simulink library "PESRC01MSEREF"  (R2014b)
settings: Solver=ode45  StartTime=0.0  StopTime=10.0  RelTol=1e-3
undefined symbols (not defined in the file): errordlg
libraries: simulink x27
settings Model: Creator=vda2sh  LastModifiedBy=RUS1COB

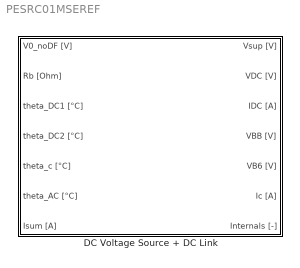
== system PESRC01MSEREF ==
  DC Voltage Source + DC Link : Subsystem  Tag=PESRC01MSEREF  mask(PESRC01MSEREF){Lb=5e-6, Cb=1, RDC120=5e-3, alphaDC1=0, RDC220=1e-3, alphaDC2=0, LDC2=4e-5, C=600e-6, Rc20=1e-3, alphac=0, RAC20=1e-3, alphaAC=0, IDC_init=0, qDC_init=0, Vc_init=0}
      mask prompts: Lb "DC voltage source internal inductance [H]"; Cb "DC voltage source capacity [Ah]"; RDC120 "Wire harness resistance at 20°C [Ohm]"; alphaDC1 "Thermal coefficient of wire harness resistance [1/K]"; RDC220 "Power net resistance at 20°C [Ohm]"; alphaDC2 "Thermal coefficient of power net resistance [1/K]"; LDC2 "Power net inductance [H]"; C "DC-link capacitor [F]"; Rc20 "DC-link resistance at 20°C [Ohm]"; alphac "Thermal coefficient of DC-link resistance [1/K]"; RAC20 "Cable resistance between DC-link and drive at 20°C [Ohm]"; alphaAC "Thermal coefficient of cable resistance between DC-link and drive [1/K]"; IDC_init "Initial DC voltage source current (case Lb+LDC2>0) [A]"; qDC_init "Initial DC voltage source charge [C]"; Vc_init "Initial DC-link capacitor voltage [V]"
      mask help:
      | PESRC01MSEREF - DC Voltage Source and DC-Link Model
      |
      | This is a model of a DC voltage source connected a DC-link considering simple wire harness and power net effects.
      settings: AttributesFormatString=<%<Tag>>
      mask Help: eval('show_docs_mseref_powerelectronics(''PESRC01MSEREF'')')
      mask Display:
      | image(imread('PESRC01MSEREF.png'),[0.25, 0.25, 0.6, 0.6]);
      | text(0.6,0.15, 'MSE')
      | port_label('input',1,'V0_NoDF [V]')
      | port_label('input',2,'Rb [Ohm]')
      | port_label('input',3,'theta_DC1 [°C]')
      | port_label('input',4,'theta_DC2 [°C]')
      | port_label('input',5,'theta_c [°C]')
      | port_label('input',6,'theta_AC [°C]')
      | port_label('input',7,'Isum [A]')
      | port_label('output',1,'Vsup [V]')
      | port_label('output',2,'VDC [V]')
      | port_label('output',3,'IDC [A]')
      | port_label('output',4,'VBB [V]')
      | port_label('output',5,'VB6 [V]')
      | port_label('output',6,'Ic [A]')
      | port_label('output',7,'Internals')

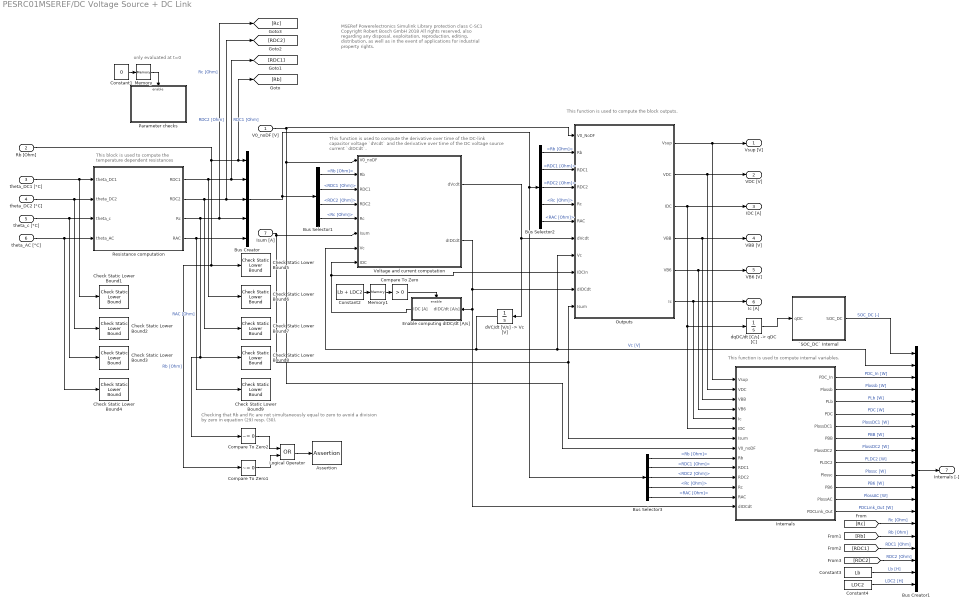
== system PESRC01MSEREF/DC Voltage Source + DC Link ==
  note: Checking that Rb and Rc are not simultaneously equal to zero to avoid
      | a division by zero in equation (29) resp. (30).
  note: This function is used to compute internal variables.
  note: This function is used to compute the block outputs.
  note: This function is used to compute the derivative over time
      | of the DC-link capacitor voltage `dVcdt`
      | and the derivative over time of the DC voltage source current `dIDCdt`.
  note: This block is used to compute
      | the temperature dependent resistances
  note: MSERef Powerelectronics Simulink Library
      | protection class C-SC1
      |
      | Copyright Robert Bosch GmbH 2018
      |
      | All rights reserved, also regarding any disposal, exploitation,
      | reproduction, editing, distribution, as well as in the event of
      | applications for industrial property rights.
  note: only evaluated at t=0
  V0_noDF [V] : Inport
  Rb [Ohm] : Inport  Port=2
  theta_DC1 [°C] : Inport  Port=3
  theta_DC2 [°C] : Inport  Port=4
  theta_c [°C] : Inport  Port=5
  theta_AC [°C] : Inport  Port=6
  Isum [A] : Inport  Port=7
  Assertion : Assertion  AssertionFailFcn=errordlg('ERROR: `DC voltage source internal resistance` Rb and `DC-link resistance`Rc(theta_c) are simultaneously equal to zero.')
  Bus Creator : BusCreator  Inputs=5
  Bus Creator1 : BusCreator  Inputs=20
  Bus Selector1 : BusSelector  OutputSignals=Rb [Ohm],RDC1 [Ohm],RDC2 [Ohm],Rc [Ohm]
  Bus Selector2 : BusSelector  OutputSignals=Rb [Ohm],RDC1 [Ohm],RDC2 [Ohm],Rc [Ohm],RAC [Ohm]
  Bus Selector3 : BusSelector  OutputSignals=Rb [Ohm],RDC1 [Ohm],RDC2 [Ohm],Rc [Ohm],RAC [Ohm]
  Check Static Lower Bound1 : simulink/Model Verification/Check Static  Lower Bound  Description=-273.15 < u  min=-273.15  min_included=off  enabled=on  callback=errordlg('Input `Wire harness temperature` theta_DC1 lower or equal to -273.15°C.')  stopWhenAssertionFail=on  export=off  icon=graphic
  Check Static Lower Bound2 : simulink/Model Verification/Check Static  Lower Bound  Description=-273.15 < u  min=-273.15  min_included=off  enabled=on  callback=errordlg('Input `Power net temperature` theta_DC2 lower or equal to -273.15°C.')  stopWhenAssertionFail=on  export=off  icon=graphic
  Check Static Lower Bound3 : simulink/Model Verification/Check Static  Lower Bound  Description=-273.15 < u  min=-273.15  min_included=off  enabled=on  callback=errordlg('Input `DC-link temperature` theta_c lower or equal to -273.15°C.')  stopWhenAssertionFail=on  export=off  icon=graphic
  Check Static Lower Bound4 : simulink/Model Verification/Check Static  Lower Bound  Description=-273.15 < u  min=-273.15  min_included=off  enabled=on  callback=errordlg('Input `Cable (between DC-link and drive) temperature` theta_AC lower or equal to -273.15°C.')  stopWhenAssertionFail=on  export=off  icon=graphic
  Check Static Lower Bound5 : simulink/Model Verification/Check Static  Lower Bound  Description=0 <= u  min=0  min_included=on  enabled=on  callback=errordlg('ERROR: `DC voltage source internal resistance` Rb is lower than zero.')  stopWhenAssertionFail=on  export=off  icon=graphic
  Check Static Lower Bound6 : simulink/Model Verification/Check Static  Lower Bound  Description=0 <= u  min=0  min_included=on  enabled=on  callback=errordlg('ERROR: `Wire harness resistance` RDC1(theta_DC1) is lower than zero.')  stopWhenAssertionFail=on  export=off  icon=graphic
  Check Static Lower Bound7 : simulink/Model Verification/Check Static  Lower Bound  Description=0 <= u  min=0  min_included=on  enabled=on  callback=errordlg('ERROR: `Power net resistance`RDC2(theta_DC2) is lower than zero.')  stopWhenAssertionFail=on  export=off  icon=graphic
  Check Static Lower Bound8 : simulink/Model Verification/Check Static  Lower Bound  Description=0 <= u  min=0  min_included=on  enabled=on  callback=errordlg('ERROR: `DC-link resistance`Rc(theta_c) is lower than zero.')  stopWhenAssertionFail=on  export=off  icon=graphic
  Check Static Lower Bound9 : simulink/Model Verification/Check Static  Lower Bound  Description=0 <= u  min=0  min_included=on  enabled=on  callback=errordlg('ERROR: `Cable resistance between DC-link and drive`RAC(theta_AC) is lower than zero.')  stopWhenAssertionFail=on  export=off  icon=graphic
  Compare To Zero : simulink/Logic and Bit Operations/Compare To Zero  relop=>  OutDataTypeStr=boolean
  Compare To Zero1 : simulink/Logic and Bit Operations/Compare To Zero  relop=~=  OutDataTypeStr=boolean
  Compare To Zero2 : simulink/Logic and Bit Operations/Compare To Zero  relop=~=  OutDataTypeStr=boolean
  Constant1 : Constant  Value=0
  Constant2 : Constant  Value=Lb + LDC2
  Constant3 : Constant  Value=Lb
  Constant4 : Constant  Value=LDC2
  Enable computing dIDC/dt [A/s] : Subsystem  TreatAsAtomicUnit=on
  Internals : MATLAB Function  TreatAsAtomicUnit=on
  Logical Operator : Logic  Operator=OR  AllPortsSameDT=off  OutDataTypeStr=boolean
  Memory : Memory  X0=1
  Memory1 : Memory  X0=1
  Outputs : MATLAB Function  TreatAsAtomicUnit=on
  Parameter checks : Subsystem
  Resistance computation : MATLAB Function  TreatAsAtomicUnit=on
  Voltage and current computation : MATLAB Function  TreatAsAtomicUnit=on
  `SOC_DC` Internal : MATLAB Function  TreatAsAtomicUnit=on
  "dVC/dt [V/s] -> Vc [V]" : Integrator  InitialCondition=Vc_init
  "dqDC/dt [C/s] -> qDC [C]" : Integrator  InitialCondition=qDC_init
  Vsup [V] : Outport
  VDC [V] : Outport  Port=2
  IDC [A] : Outport  Port=3
  VBB [V] : Outport  Port=4
  VB6 [V] : Outport  Port=5
  Ic [A] : Outport  Port=6
  Internals [-] : Outport  Port=7
  wires:
  Internals/7(PlossDC2) -> Bus Creator1/9  "PlossDC2 [W]"
  Internals/5(PlossDC1) -> Bus Creator1/7  "PlossDC1 [W]"
  Internals/9(Plossc) -> Bus Creator1/11  "Plossc [W]"
  Internals/3(PLb) -> Bus Creator1/5  "PLb [W]"
  Internals/11(PlossAC) -> Bus Creator1/13  "PlossAC [W]"
  Internals/12(PDCLink_Out) -> Bus Creator1/14  "PDCLink_Out [W]"
  Internals/8(PLDC2) -> Bus Creator1/10  "PLDC2 [W]"
  Internals/2(Plossb) -> Bus Creator1/4  "Plossb [W]"
  Internals/1(PDC_In) -> Bus Creator1/3  "PDC_In [W]"
  Bus Creator1/1 -> Internals [-]/1
  "dVC/dt [V/s] -> Vc [V]"/1 -> Voltage and current computation/7(Vc), Outputs/8(Vc), Bus Creator1/2  "Vc [V]"
  Bus Selector2/4 -> Outputs/5(Rc)  "<Rc [Ohm]>"
  Bus Selector2/2 -> Outputs/3(RDC1)  "<RDC1 [Ohm]>"
  Bus Selector3/2 -> Internals/10(RDC1)  "<RDC1 [Ohm]>"
  Bus Selector3/4 -> Internals/12(Rc)  "<Rc [Ohm]>"
  Bus Selector3/1 -> Internals/9(Rb)  "<Rb [Ohm]>"
  Bus Selector3/5 -> Internals/13(RAC)  "<RAC [Ohm]>"
  Bus Selector3/3 -> Internals/11(RDC2)  "<RDC2 [Ohm]>"
  Bus Selector2/1 -> Outputs/2(Rb)  "<Rb [Ohm]>"
  Bus Selector1/4 -> Voltage and current computation/5(Rc)  "<Rc [Ohm]>"
  Bus Selector1/3 -> Voltage and current computation/4(RDC2)  "<RDC2 [Ohm]>"
  Bus Selector1/2 -> Voltage and current computation/3(RDC1)  "<RDC1 [Ohm]>"
  Bus Selector1/1 -> Voltage and current computation/2(Rb)  "<Rb [Ohm]>"
  Bus Creator/1 -> Bus Selector1/1, Bus Selector3/1, Bus Selector2/1
  Resistance computation/4(RAC) -> Check Static Lower Bound9/1, Bus Creator/5  "RAC [Ohm]"
  Resistance computation/1(RDC1) -> Check Static Lower Bound6/1, [RDC1], Bus Creator/2  "RDC1 [Ohm]"
  Resistance computation/2(RDC2) -> Check Static Lower Bound7/1, [RDC2], Bus Creator/3  "RDC2 [Ohm]"
  theta_AC [°C]/1 -> Check Static Lower Bound4/1, Resistance computation/4(theta_AC)
  theta_c [°C]/1 -> Check Static Lower Bound3/1, Resistance computation/3(theta_c)
  theta_DC2 [°C]/1 -> Check Static Lower Bound2/1, Resistance computation/2(theta_DC2)
  theta_DC1 [°C]/1 -> Check Static Lower Bound1/1, Resistance computation/1(theta_DC1)
  Outputs/1(Vsup) -> Internals/1(Vsup), Vsup [V]/1
  Voltage and current computation/1(dVcdt) -> Outputs/7(dVcdt), "dVC/dt [V/s] -> Vc [V]"/1
  Isum [A]/1 -> Outputs/11(Isum), Internals/7(Isum), Voltage and current computation/6(Isum)
  Voltage and current computation/2(dIDCdt) -> Enable computing dIDC/dt [A/s]/1(dIDC/dt [A/s]), Internals/14(dIDCdt), Outputs/10(dIDCdt)
  Outputs/2(VDC) -> VDC [V]/1, Internals/2(VDC)
  Outputs/3(IDC) -> IDC [A]/1, Internals/6(IDC), "dqDC/dt [C/s] -> qDC [C]"/1
  Outputs/4(VBB) -> Internals/3(VBB), VBB [V]/1
  Outputs/5(VB6) -> Internals/4(VB6), VB6 [V]/1
  Outputs/6(Ic) -> Internals/5(Ic), Ic [A]/1
  Constant1/1 -> Memory/1
  Memory/1 -> Parameter checks/Enable
  V0_noDF [V]/1 -> Voltage and current computation/1(V0_noDF), Internals/8(V0_noDF), Outputs/1(V0_NoDF)
  Internals/10(PB6) -> Bus Creator1/12  "PB6 [W]"
  Internals/6(PBB) -> Bus Creator1/8  "PBB [W]"
  Internals/4(PDC) -> Bus Creator1/6  "PDC [W]"
  Enable computing dIDC/dt [A/s]/1(IDC [A]) -> Outputs/9(IDCIn), Voltage and current computation/8(IDC)
  Bus Selector2/5 -> Outputs/6(RAC)  "<RAC [Ohm]>"
  Bus Selector2/3 -> Outputs/4(RDC2)  "<RDC2 [Ohm]>"
  Compare To Zero/1 -> Enable computing dIDC/dt [A/s]/Enable
  Memory1/1 -> Compare To Zero/1
  Constant2/1 -> Memory1/1
  Compare To Zero2/1 -> Logical Operator/1
  Compare To Zero1/1 -> Logical Operator/2
  Logical Operator/1 -> Assertion/1
  `SOC_DC` Internal/1(SOC_DC) -> Bus Creator1/1  "SOC_DC [-]"
  "dqDC/dt [C/s] -> qDC [C]"/1 -> `SOC_DC` Internal/1(qDC)
  Resistance computation/3(Rc) -> Compare To Zero2/1, Check Static Lower Bound8/1, [Rc], Bus Creator/4  "Rc [Ohm]"
  Rb [Ohm]/1 -> Compare To Zero1/1, Check Static Lower Bound5/1, [Rb], Bus Creator/1  "Rb [Ohm]"
  [Rc] -> Bus Creator1/15  "Rc [Ohm]"
  [Rb] -> Bus Creator1/16  "Rb [Ohm]"
  [RDC1] -> Bus Creator1/17  "RDC1 [Ohm]"
  [RDC2] -> Bus Creator1/18  "RDC2 [Ohm]"
  Constant3/1 -> Bus Creator1/19  "Lb [H]"
  Constant4/1 -> Bus Creator1/20  "LDC2 [H]"

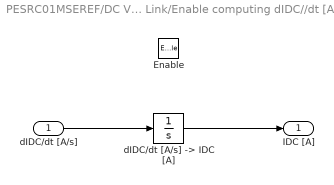
== system PESRC01MSEREF/DC Voltage Source + DC Link/Enable computing dIDC//dt [A//s] ==
  dIDC/dt [A/s] : Inport
  Enable : EnablePort
  "dIDC/dt [A/s] -> IDC [A]" : Integrator  InitialCondition=IDC_init
  IDC [A] : Outport
  wires:
  dIDC/dt [A/s]/1 -> "dIDC/dt [A/s] -> IDC [A]"/1
  "dIDC/dt [A/s] -> IDC [A]"/1 -> IDC [A]/1

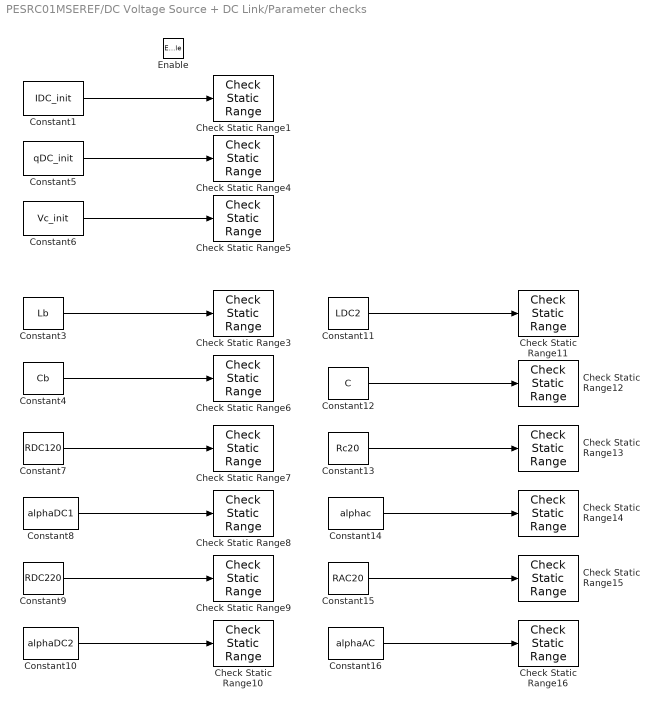
== system PESRC01MSEREF/DC Voltage Source + DC Link/Parameter checks ==
  Enable : EnablePort  ZeroCross=off
  Check Static Range1 : simulink/Model Verification/Check  Static Range  Description=-1e9 <= u < 1e9  max=1e9  max_included=off  min=-1e9  min_included=on  enabled=on  callback=errordlg('Parameter `Initial DC voltage source current` IDC_init outside boundary [-1e9, 1e9] A.')  stopWhenAssertionFail=on  export=off  icon=graphic
  Check Static Range10 : simulink/Model Verification/Check  Static Range  Description=0 <= u <= 1  max=1  max_included=on  min=0  min_included=on  enabled=on  callback=errordlg('Parameter `Thermal coefficient of power net resistance` alphaDC1 outside boundary [0, 1] 1/K.')  stopWhenAssertionFail=on  export=off  icon=graphic
  Check Static Range11 : simulink/Model Verification/Check  Static Range  Description=0 <= u <= 10  max=10  max_included=on  min=0  min_included=on  enabled=on  callback=errordlg('Parameter `Power net inductance` LDC2 outside boundary [0, 10] H.')  stopWhenAssertionFail=on  export=off  icon=graphic
  Check Static Range12 : simulink/Model Verification/Check  Static Range  Description=0 <= u <= 1e3  max=1e3  max_included=on  min=0  min_included=on  enabled=on  callback=errordlg('Parameter `DC-link capacitor` C outside boundary [0, 1e3] F.')  stopWhenAssertionFail=on  export=off  icon=graphic
  Check Static Range13 : simulink/Model Verification/Check  Static Range  Description=0 <= u <= 1e9  max=1e9  max_included=on  min=0  min_included=on  enabled=on  callback="errordlg('Parameter `DC-link resistance  at 20°C` Rc20 outside boundary ]0, 1e9] Ohm.')"  stopWhenAssertionFail=on  export=off  icon=graphic
  Check Static Range14 : simulink/Model Verification/Check  Static Range  Description=0 <= u <= 1  max=1  max_included=on  min=0  min_included=on  enabled=on  callback=errordlg('Parameter `Thermal coefficient of DC-link resistance` alphac outside boundary [0, 1] 1/K.')  stopWhenAssertionFail=on  export=off  icon=graphic
  Check Static Range15 : simulink/Model Verification/Check  Static Range  Description=0 <= u <= 1e9  max=1e9  max_included=on  min=0  min_included=on  enabled=on  callback=errordlg('Parameter `Cable resistance between DC-link and drive at 20°C` RAC20 outside boundary [0, 1e9] Ohm.')  stopWhenAssertionFail=on  export=off  icon=graphic
  Check Static Range16 : simulink/Model Verification/Check  Static Range  Description=0 <= u <= 1  max=1  max_included=on  min=0  min_included=on  enabled=on  callback=errordlg('Parameter `Thermal coefficient of cable resistance between DC-link and drive` alphaAC outside boundary [0, 1] 1/K.')  stopWhenAssertionFail=on  export=off  icon=graphic
  Check Static Range3 : simulink/Model Verification/Check  Static Range  Description=0 <= u <= 10  max=10  max_included=on  min=0  min_included=on  enabled=on  callback=errordlg('Parameter `DC voltage source internal inductance` Lb outside boundary [0, 10] H.')  stopWhenAssertionFail=on  export=off  icon=graphic
  Check Static Range4 : simulink/Model Verification/Check  Static Range  Description=-1e9 <= u < 1e9  max=1e9  max_included=off  min=-1e9  min_included=on  enabled=on  callback=errordlg('Parameter `Initial DC voltage source charge` qDC_init outside boundary [-1e9, 1e9] C.')  stopWhenAssertionFail=on  export=off  icon=graphic
  Check Static Range5 : simulink/Model Verification/Check  Static Range  Description=-1e9 <= u < 1e9  max=1e9  max_included=off  min=-1e9  min_included=on  enabled=on  callback=errordlg('Parameter `Initial DC-link capacitor voltage` Vc_init outside boundary [-1e9, 1e9] V.')  stopWhenAssertionFail=on  export=off  icon=graphic
  Check Static Range6 : simulink/Model Verification/Check  Static Range  Description=0 <= u <= 10  max=10  max_included=on  min=0  min_included=on  enabled=on  callback=errordlg('Parameter `DC voltage source capacity` Cb outside boundary [0, 10] Ah.')  stopWhenAssertionFail=on  export=off  icon=graphic
  Check Static Range7 : simulink/Model Verification/Check  Static Range  Description=0 <= u <= 1e9  max=1e9  max_included=on  min=0  min_included=on  enabled=on  callback="errordlg('Parameter `Wire harness resistance  at 20°C` RDC120 outside boundary [0, 1e9] Ohm.')"  stopWhenAssertionFail=on  export=off  icon=graphic
  Check Static Range8 : simulink/Model Verification/Check  Static Range  Description=0 <= u <= 1  max=1  max_included=on  min=0  min_included=on  enabled=on  callback=errordlg('Parameter `Thermal coefficient of wire harness resistance` alphaDC1 outside boundary [0, 1] 1/K.')  stopWhenAssertionFail=on  export=off  icon=graphic
  Check Static Range9 : simulink/Model Verification/Check  Static Range  Description=0 <= u <= 1e9  max=1e9  max_included=on  min=0  min_included=on  enabled=on  callback=errordlg('Parameter `Power net resistance at 20°C` RDC220 outside boundary [0, 1e9] Ohm.')  stopWhenAssertionFail=on  export=off  icon=graphic
  Constant1 : Constant  Value=IDC_init
  Constant10 : Constant  Value=alphaDC2
  Constant11 : Constant  Value=LDC2
  Constant12 : Constant  Value=C
  Constant13 : Constant  Value=Rc20
  Constant14 : Constant  Value=alphac
  Constant15 : Constant  Value=RAC20
  Constant16 : Constant  Value=alphaAC
  Constant3 : Constant  Value=Lb
  Constant4 : Constant  Value=Cb
  Constant5 : Constant  Value=qDC_init
  Constant6 : Constant  Value=Vc_init
  Constant7 : Constant  Value=RDC120
  Constant8 : Constant  Value=alphaDC1
  Constant9 : Constant  Value=RDC220
  wires:
  Constant1/1 -> Check Static Range1/1
  Constant5/1 -> Check Static Range4/1
  Constant6/1 -> Check Static Range5/1
  Constant3/1 -> Check Static Range3/1
  Constant4/1 -> Check Static Range6/1
  Constant7/1 -> Check Static Range7/1
  Constant8/1 -> Check Static Range8/1
  Constant9/1 -> Check Static Range9/1
  Constant10/1 -> Check Static Range10/1
  Constant11/1 -> Check Static Range11/1
  Constant12/1 -> Check Static Range12/1
  Constant13/1 -> Check Static Range13/1
  Constant14/1 -> Check Static Range14/1
  Constant15/1 -> Check Static Range15/1
  Constant16/1 -> Check Static Range16/1

== matlab function PESRC01MSEREF/DC Voltage Source + DC Link/Resistance computation ==
  data: theta_DC1 input; theta_DC2 input; theta_c input; theta_AC input; RDC120 parameter; alphaDC1 parameter; RDC220 parameter; alphaDC2 parameter; Rc20 parameter; alphac parameter; RDC1 output; RDC2 output; Rc output; RAC20 parameter; alphaAC parameter; RAC output
function [RDC1, RDC2, Rc, RAC] = fcn_Resistance(theta_DC1, theta_DC2, theta_c, theta_AC, RDC120, alphaDC1, RDC220, alphaDC2, Rc20, alphac, RAC20, alphaAC)
% This function is used to compute the temperature dependent resistances
%
%  MSERef Powerelectronics Simulink Library 
%  protection class C-SC1
%
%  Copyright Robert Bosch GmbH 2018
%
%  All rights reserved, also regarding any disposal, exploitation,
%  reproduction, editing, distribution, as well as in the event of
%  applications for industrial property rights.

  
%#codegen

RDC1 = RDC120*( 1 + alphaDC1* (theta_DC1 - 20) );% Implementing equation (13)

RDC2 = RDC220*( 1 + alphaDC2* (theta_DC2 - 20) );% Implementing equation (17)

Rc = Rc20*( 1 + alphac* (theta_c - 20) );% Implementing equation (21)

RAC = RAC20*( 1 + alphaAC* (theta_AC - 20) );% Implementing equation (24)

== matlab function PESRC01MSEREF/DC Voltage Source + DC Link/Internals ==
  data: Vsup input; VDC input; VBB input; VB6 input; Ic input; IDC input; Isum input; V0_noDF input; Rb input; Lb parameter; RDC1 input; RDC2 input; LDC2 parameter; Rc input; RAC input; dIDCdt input; PDC_In output; Plossb output; PLb output; PDC output; PlossDC1 output; PBB output; PlossDC2 output; PLDC2 output; Plossc output; PB6 output; PlossAC output; PDCLink_Out output
function [PDC_In, Plossb, PLb, PDC, PlossDC1, PBB, PlossDC2, PLDC2, Plossc, PB6, PlossAC, PDCLink_Out] = fcn_Internals(Vsup, VDC, VBB, VB6, Ic, IDC, Isum, V0_noDF, Rb, Lb, RDC1, RDC2, LDC2, Rc, RAC, dIDCdt)
% This function is used to compute internal variables
% `PDC_In`, `Plossb`, `PLb`, `PDC`, `PlossDC1`, `PBB`, `PlossDC2`, 
% `PLDC2`, `Plossc`, `PB6`, `PlossAC`, `PDCLink_Out`.
%
%  MSERef Powerelectronics Simulink Library 
%  protection class C-SC1
%
%  Copyright Robert Bosch GmbH 2018
%
%  All rights reserved, also regarding any disposal, exploitation,
%  reproduction, editing, distribution, as well as in the event of
%  applications for industrial property rights.


% Computing `Internals` variable
PDC_In = V0_noDF*IDC; % Implementing equation (8)
Plossb = Rb*IDC^2; % Implementing equation (9)
PLb = Lb*dIDCdt*IDC; % Implementing equation (10)
PDC = VDC*IDC; % Implementing equation (11)
PlossDC1 = RDC1*IDC^2; % Implementing equation (14)
PBB = VBB*IDC; % Implementing equation (15)
PlossDC2 = RDC2*IDC^2; % Implementing equation (18)
PLDC2 = LDC2*dIDCdt*IDC; % Implementing equation (19)
Plossc = Rc*Ic^2; % Implementing equation (22)
PB6 = VB6*Isum; % Implementing equation (23)
PlossAC = RAC*Isum^2; % Implementing equation (25)
PDCLink_Out = Vsup*Isum; % Implementing equation (26)

== matlab function PESRC01MSEREF/DC Voltage Source + DC Link/`SOC_DC` Internal ==
  data: qDC input; Cb parameter; SOC_DC output
function SOC_DC = SOC_DC_Internal(qDC, Cb)
% This function is used to compute internal variable `SOC_DC`
%
%  MSERef Powerelectronics Simulink Library 
%  protection class C-SC1
%
%  Copyright Robert Bosch GmbH 2018
%
%  All rights reserved, also regarding any disposal, exploitation,
%  reproduction, editing, distribution, as well as in the event of
%  applications for industrial property rights.

% Computing nominal charge `qDC_Nom` of the DC voltage source
% Implementing equation (6) from `PESRC01MSEREF_details.pdf` documentation
qDC_Nom = Cb*3600;

% Computing `SOC_DC` Internal variable
SOC_DC = 1 - qDC / qDC_Nom; % Implementing equation (4) from `PESRC01MSEREF_details.pdf` documentation

== matlab function PESRC01MSEREF/DC Voltage Source + DC Link/Outputs ==
  data: Vsup output; V0_NoDF input; Rb input; Lb parameter; RDC1 input; RDC2 input; Rc input; RAC input; dVcdt input; Vc input; IDCIn input; dIDCdt input; LDC2 parameter; C parameter; Isum input; VDC output; IDC output; VBB output; VB6 output; Ic output
function [Vsup, VDC, IDC, VBB, VB6, Ic] = fcn_Outputs(V0_NoDF, Rb, Lb, RDC1, RDC2, Rc, RAC, dVcdt, Vc, IDCIn, dIDCdt, LDC2, C, Isum)
% This function is used to compute the block outputs `Vsup`, `VDC`, `IDC`, `VBB`, `VB6` and `Ic`.
%
%  MSERef Powerelectronics Simulink Library 
%  protection class C-SC1
%
%  Copyright Robert Bosch GmbH 2018
%
%  All rights reserved, also regarding any disposal, exploitation,
%  reproduction, editing, distribution, as well as in the event of
%  applications for industrial property rights.

%#codegen
coder.extrinsic('errordlg');

% Computing DC-link current `Ic` (needed to compute `IDC`)
% Implementing equation (20) from `PESRC01MSEREF_details.pdf` documentation
Ic = C*dVcdt;

% Computing DC voltage source current `IDC` (needed to compute `VDC`)
if ( Lb + LDC2 ) > 0.0
    % Implementing equation (27) from `PESRC01MSEREF_details.pdf` documentation    
    Vsup = (Rb + RDC1 + RDC2)/(Rb + RDC1 + RDC2 + Rc) * Vc ...
        + Rc/(Rb + RDC1 + RDC2 + Rc) * (V0_NoDF - (Rb + RDC1 + RDC2)*Isum - ( Lb + LDC2 )*dIDCdt ) ...
        - RAC * Isum;
    
    % if Lb + LDC2 > 0.0, `IDC` is computed from its derivative (equation (2))
    % in `Voltage and current computation` block.
    IDC = IDCIn;
    
elseif ( Lb + LDC2 ) == 0.0
    % Implementing equation (28) from `PESRC01MSEREF_details.pdf` documentation
    Vsup = (Rb + RDC1 + RDC2)/(Rb + RDC1 + RDC2 + Rc) * Vc ...
        + Rc/(Rb + RDC1 + RDC2 + Rc) * (V0_NoDF - (Rb + RDC1 + RDC2)*Isum ) ...
        - RAC * Isum;

    % Implementing equation (3) from `PESRC01MSEREF_details.pdf` documentation
    IDC = Isum + Ic;

else % ( Lb + LDC2 ) < 0.0
    Vsup = 0.0;
    IDC = 0.0;
    errordlg('ERROR: `Lb + LDC2` must be positive or equal to zero.');
end

% Computing DC-source voltage `VDC`
% Implementing equation (1) from `PESRC01MSEREF_details.pdf` documentation
VDC = V0_NoDF - Rb*IDC - Lb*dIDCdt;

% Computing voltage `VBB`
% Implementing equation (12) from `PESRC01MSEREF_details.pdf` documentation
VBB = VDC - RDC1*IDC;

% Computing voltage `VB6`
% Implementing equation (16) from `PESRC01MSEREF_details.pdf` documentation
VB6 = Vc + Rc*Ic;

== matlab function PESRC01MSEREF/DC Voltage Source + DC Link/Voltage and current computation ==
  data: V0_noDF input; Rb input; Lb parameter; RDC1 input; RDC2 input; Rc input; LDC2 parameter; C parameter; Isum input; Vc input; dVcdt output; dIDCdt output; IDC input
function [dVcdt, dIDCdt] = fcn_Voltage(V0_noDF, Rb, Lb, ...
                        RDC1, RDC2, Rc, LDC2, C, Isum, Vc, IDC)
% This function is used to compute the derivative over time 
% of the DC-link capacitor voltage `dVcdt`
% and the derivative over time of the DC voltage source current `dIDCdt`.
%
%  MSERef Powerelectronics Simulink Library 
%  protection class C-SC1
%
%  Copyright Robert Bosch GmbH 2018
%
%  All rights reserved, also regarding any disposal, exploitation,
%  reproduction, editing, distribution, as well as in the event of
%  applications for industrial property rights.

%#codegen
coder.extrinsic('errordlg');

% Computing `Vsup`, `dVcdt` and `dIDCdt according to the value of `Lb + LDC2`
if ( Lb + LDC2 ) > 0.0
    % Implementing equations (2) and (29) from `PESRC01MSEREF_details.pdf` documentation
    dIDCdt = (V0_noDF - (Rb + RDC1 + RDC2 +Rc)*IDC + Rc*Isum - Vc )/( Lb + LDC2 ); % needed by `Vsup` and `dVcdt`

    dVcdt = 1/((Rb + RDC1 + RDC2 + Rc)*C) * (V0_noDF - (Rb + RDC1 + RDC2)*Isum -( Lb + LDC2 )*dIDCdt - Vc);
   
elseif ( Lb + LDC2 ) == 0.0
    % If Lb + LDC2 = 0.0, `IDC` is computed algebraically from
    % equation (3) in `Output` block.
    dIDCdt = 0.0;
        
    % Implementing equation (30) from `PESRC01MSEREF_details.pdf` documentation
    dVcdt = 1/((Rb + RDC1 + RDC2 + Rc)*C) * (V0_noDF - (Rb + RDC1 + RDC2)*Isum - Vc);
        
else % ( Lb + LDC2 ) < 0.0
    dIDCdt = 0.0;
    dVcdt = 0.0;
    errordlg('ERROR: `Lb + LDC2` must be positive or equal to zero.');
end
